simulink model "FrequencyChecker"  (R2025a)
settings: Solver=FixedStepDiscrete  StartTime=0.0  StopTime=inf  RelTol=1e-3
undefined symbols (not defined in the file): Add, phIncr, Shift
libraries: dsphdlmathfun2 x1, dsphdlxfrm2 x1, dsphdlsigops2 x1
settings Model: SimulationMode=accelerator  Creator=gxoro  LastModifiedBy=gxoro

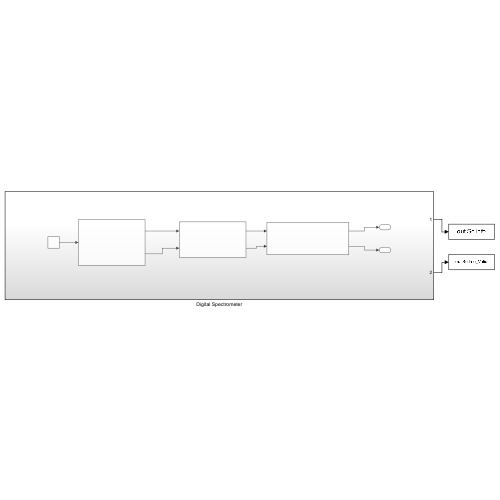
[thumbnail: Simulink's stored preview of the top-level diagram]
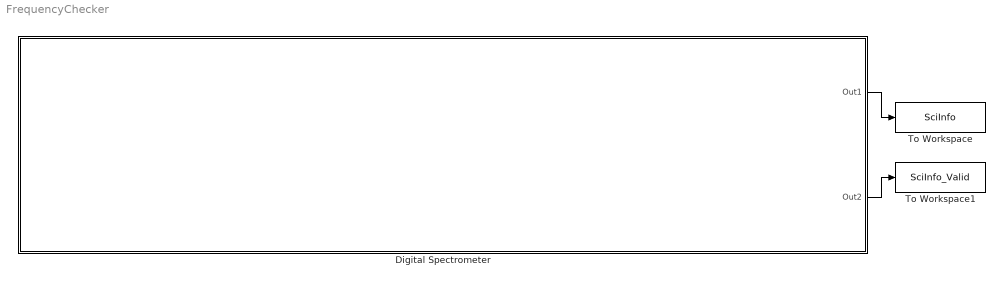
== system FrequencyChecker ==
  Digital Spectrometer : Subsystem
  To Workspace : ToWorkspace  VariableName=SciInfo  SampleTime=-1
      settings: Save2DSignal=2-D array (concatenate along first dimension)
  To Workspace1 : ToWorkspace  VariableName=SciInfo_Valid  SampleTime=-1
      settings: Save2DSignal=2-D array (concatenate along first dimension)
  wires:
  Digital Spectrometer/1(Out1) -> To Workspace/1
  Digital Spectrometer/2(Out2) -> To Workspace1/1

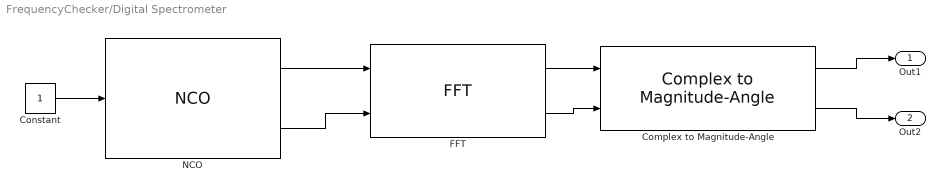
== system FrequencyChecker/Digital Spectrometer ==
  Complex to Magnitude-Angle : dsphdlmathfun2/Complex to Magnitude-Angle  NumIterationsSource=Auto  NumIterations=10  OutputFormat=Magnitude  AngleFormat=Normalized  ScaleOutput=on  ScalingMethod=Shift-Add  SimulateUsing=Code generation
  Constant : Constant  OutDataTypeStr=boolean  SampleTime=1
  FFT : dsphdlxfrm2/FFT  Architecture=Streaming Radix 2^2  FFTLengthSource=Property  FFTLength=FFT  FFTLengthMax=1024  ComplexMultiplication=Use 4 multipliers and 2 adders  BitReversedOutput=off  BitReversedInput=off  Normalize=off  SimulateUsing=Code generation  RoundingMethod=Floor  ResetInputPort=off  StartOutputPort=off  EndOutputPort=off
  NCO : dsphdlsigops2/NCO  PhaseIncrementSource=Property  PhaseIncrement=phIncr(5)  PhaseOffsetSource=Property  PhaseOffset=phOff  DitherSource=Property  NumDitherBits=4  SamplesPerFrame=1  LUTCompress=off  ResetAction=off  Waveform=Sine  PhasePort=off  SimulateUsing=Code generation  AccumulatorWL=N  PhaseQuantization=on  NumQuantizerAccumulatorBits=Q  OutputDataType=Binary point scaling  OutputWL=16  OutputFL=14
      settings: LibrarySourceBlock=dsphdlsrcs2/NCO
  Out1 : Outport
  Out2 : Outport  Port=2
  wires:
  FFT/1 -> Complex to Magnitude-Angle/1
  NCO/2 -> FFT/2
  Complex to Magnitude-Angle/2 -> Out2/1
  Constant/1 -> NCO/1
  NCO/1 -> FFT/1
  FFT/2 -> Complex to Magnitude-Angle/2
  Complex to Magnitude-Angle/1 -> Out1/1
